simulink model "zad2"  (R2020b)
settings: Solver=FixedStepDiscrete  StartTime=0.0  StopTime=0  RelTol=1e-3
undefined symbols (not defined in the file): magnitude
libraries: CPOiS_SourcesSinks x9, CPOiS_Edges x3, CPOiS_DataManipulation_DataTypeConversion x3, CPOiS_DataManipulation x2, CPOiS_LinearTransforms x2, CPOiS_General x1, simulink_extras x1
settings Model: Creator=jrybarz  LastModifiedBy=jrybarz

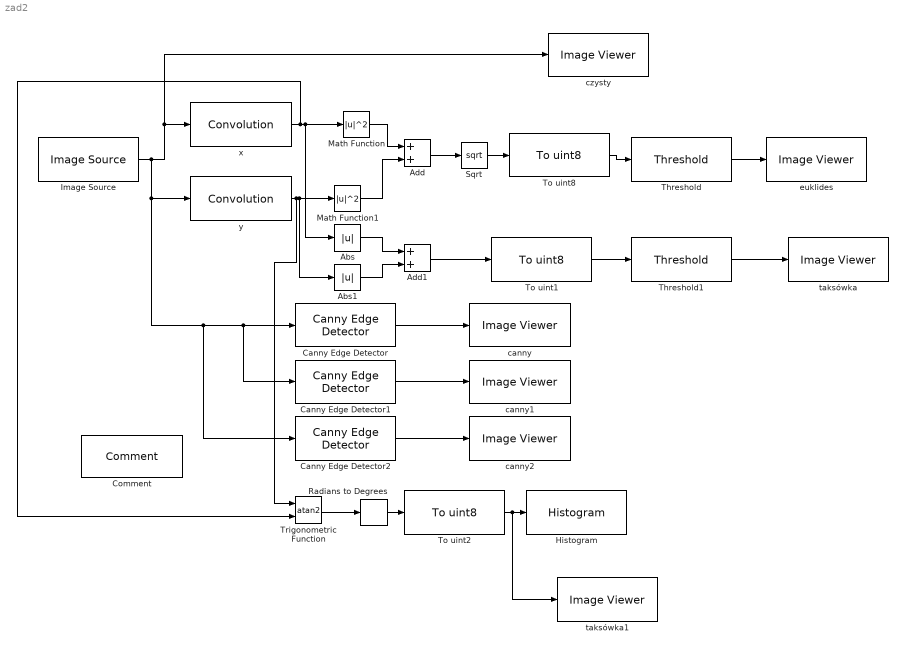
== system zad2 ==
  Abs : Abs
  Abs1 : Abs
  Add : Sum
  Add1 : Sum
  Canny Edge Detector : CPOiS_Edges/Canny Edge Detector  LowThresh=0  HighThresh=100
      settings: SourceProductName=CPOiS - Digital image and signal processing
  Canny Edge Detector1 : CPOiS_Edges/Canny Edge Detector  LowThresh=0  HighThresh=200
      settings: SourceProductName=CPOiS - Digital image and signal processing
  Canny Edge Detector2 : CPOiS_Edges/Canny Edge Detector  LowThresh=80  HighThresh=100
      settings: SourceProductName=CPOiS - Digital image and signal processing
  Comment : CPOiS_General/Comment
      settings: SourceProductName=CPOiS - Digital image and signal processing
  Histogram : CPOiS_SourcesSinks/Histogram
      settings: SourceProductName=CPOiS - Digital image and signal processing
  Image Source : CPOiS_SourcesSinks/Image Source  FileSelection=gull.png
      settings: SourceProductName=CPOiS - Digital image and signal processing
  Math Function : Math  Operator=magnitude^2  SaturateOnIntegerOverflow=on
  Math Function1 : Math  Operator=magnitude^2  SaturateOnIntegerOverflow=on
  Radians to Degrees : simulink_extras/Transformations/Radians to Degrees
  Sqrt : Sqrt  SaturateOnIntegerOverflow=on
  Threshold : CPOiS_DataManipulation/Threshold  Threshold=127
      settings: SourceProductName=CPOiS - Digital image and signal processing
  Threshold1 : CPOiS_DataManipulation/Threshold  Threshold=127
      settings: SourceProductName=CPOiS - Digital image and signal processing
  To uint1 : CPOiS_DataManipulation_DataTypeConversion/To uint8
      settings: SourceProductName=CPOiS - Digital image and signal processing
  To uint2 : CPOiS_DataManipulation_DataTypeConversion/To uint8
      settings: SourceProductName=CPOiS - Digital image and signal processing
  To uint8 : CPOiS_DataManipulation_DataTypeConversion/To uint8
      settings: SourceProductName=CPOiS - Digital image and signal processing
  Trigonometric Function : Trigonometry  Operator=atan2
  canny : CPOiS_SourcesSinks/Image Viewer
      settings: SourceProductName=CPOiS - Digital image and signal processing
  canny1 : CPOiS_SourcesSinks/Image Viewer
      settings: SourceProductName=CPOiS - Digital image and signal processing
  canny2 : CPOiS_SourcesSinks/Image Viewer
      settings: SourceProductName=CPOiS - Digital image and signal processing
  czysty : CPOiS_SourcesSinks/Image Viewer
      settings: SourceProductName=CPOiS - Digital image and signal processing
  euklides : CPOiS_SourcesSinks/Image Viewer
      settings: SourceProductName=CPOiS - Digital image and signal processing
  taksówka : CPOiS_SourcesSinks/Image Viewer
      settings: SourceProductName=CPOiS - Digital image and signal processing
  taksówka1 : CPOiS_SourcesSinks/Image Viewer
      settings: SourceProductName=CPOiS - Digital image and signal processing
  x : CPOiS_LinearTransforms/Convolution  ConvolutionMatrix=[-1,0,1;-2,0,2;-1,0,1]
      settings: SourceProductName=CPOiS - Digital image and signal processing
  y : CPOiS_LinearTransforms/Convolution  ConvolutionMatrix=[-1,-2,-1;0,0,0;1,2,1]
      settings: SourceProductName=CPOiS - Digital image and signal processing
  wires:
  x/1 -> Trigonometric Function/2, Abs/1, Math Function/1
  y/1 -> Trigonometric Function/1, Abs1/1, Math Function1/1
  Math Function/1 -> Add/1
  Math Function1/1 -> Add/2
  Add/1 -> Sqrt/1
  Image Source/1 -> Canny Edge Detector2/1, Canny Edge Detector1/1, Canny Edge Detector/1, y/1, czysty/1, x/1
  Threshold/1 -> euklides/1
  Sqrt/1 -> To uint8/1
  To uint8/1 -> Threshold/1
  Canny Edge Detector/1 -> canny/1
  Abs/1 -> Add1/1
  Abs1/1 -> Add1/2
  Add1/1 -> To uint1/1
  To uint1/1 -> Threshold1/1
  Threshold1/1 -> taksówka/1
  Trigonometric Function/1 -> Radians to Degrees/1
  Radians to Degrees/1 -> To uint2/1
  To uint2/1 -> taksówka1/1, Histogram/1
  Canny Edge Detector1/1 -> canny1/1
  Canny Edge Detector2/1 -> canny2/1
